simulink model "Proyecto_labII_V1"  (R2025a)
settings: Solver=VariableStepAuto  StartTime=0.0  StopTime=10  RelTol=1e-3
settings Model: Creator=juand  LastModifiedBy=juand

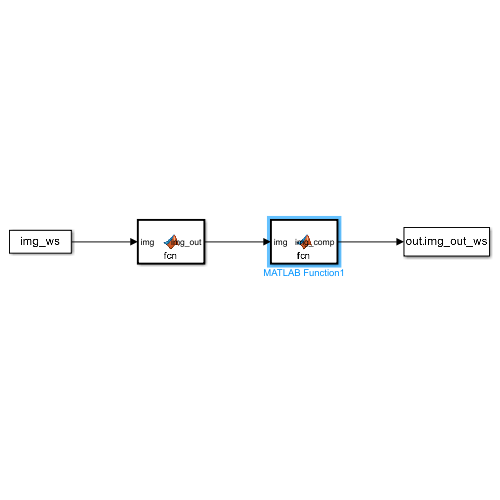
[thumbnail: Simulink's stored preview of the top-level diagram]
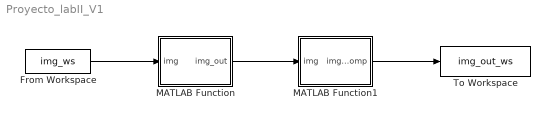
== system Proyecto_labII_V1 ==
  From Workspace : FromWorkspace  VariableName=img_ws  SampleTime=-1
  MATLAB Function : MATLAB Function  TreatAsAtomicUnit=on
  MATLAB Function1 : MATLAB Function  TreatAsAtomicUnit=on
  To Workspace : ToWorkspace  VariableName=img_out_ws  SaveFormat=Timeseries  SampleTime=-1
  wires:
  From Workspace/1 -> MATLAB Function/1(img)
  MATLAB Function/1(img_out) -> MATLAB Function1/1(img)
  MATLAB Function1/1(img_comp) -> To Workspace/1

== matlab function Proyecto_labII_V1/MATLAB Function ==
  data: img input; img_out output
function img_out = fcn(img)
%#codegen
% Procesamiento básico de imagen RGB en Simulink

% Asegurar tipo double para procesamiento
img_d = double(img);

% Verificar que sea imagen RGB
if size(img_d,3) ~= 3
    error('La imagen no es RGB');
end

% Conversión a escala de grises (luminancia)
img_gray = 0.2989 * img_d(:,:,1) + ...
           0.5870 * img_d(:,:,2) + ...
           0.1140 * img_d(:,:,3);

% Volver a uint8 para visualización
img_out = uint8(img_gray);

end

== matlab function Proyecto_labII_V1/MATLAB Function1 ==
  data: img input; img_comp output
function img_comp = fcn(img)

img = double(img);

[m,n,channels] = size(img);

m2 = floor(m/2)*2;
n2 = floor(n/2)*2;

img = img(1:m2,1:n2,:);

img_comp = zeros(m2,n2,channels);

T = 15;

for c = 1:channels
    
    I = img(:,:,c);

    L = (I(:,1:2:n2) + I(:,2:2:n2))/2;
    H = (I(:,1:2:n2) - I(:,2:2:n2))/2;

    LL = (L(1:2:m2,:) + L(2:2:m2,:))/2;
    LH = (L(1:2:m2,:) - L(2:2:m2,:))/2;
    HL = (H(1:2:m2,:) + H(2:2:m2,:))/2;
    HH = (H(1:2:m2,:) - H(2:2:m2,:))/2;

    LH(abs(LH) < T) = 0;
    HL(abs(HL) < T) = 0;
    HH(abs(HH) < T) = 0;

    % organizar subbandas como en la teoria Haar

    img_comp(:,:,c) = [LL HL; LH HH];

end

end
